simulink model "test_turb_sf9"  (R2013b)
settings: Solver=FixedStepDiscrete  StartTime=0.0  StopTime=15  FixedStep=0.005  RelTol=1e-3
libraries: simulink x1
settings Model: Creator=HSidaoui  LastModifiedBy=AGSilva
settings OptimizationCC: ExpressionDepthLimit=2147483647
settings DebuggingCC: StateNameClashWarn=warning

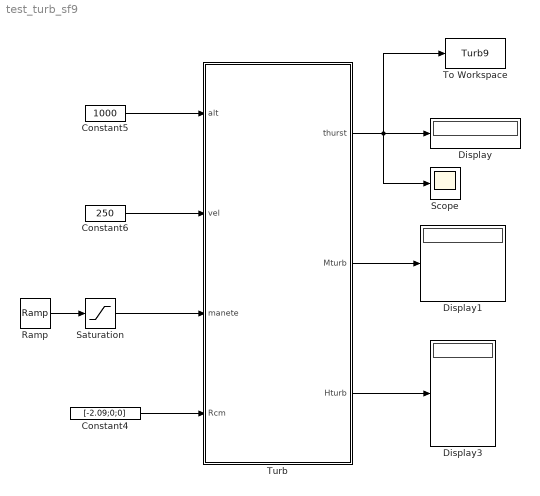
== system test_turb_sf9 ==
  Constant4 : Constant  Value=[-2.09;0;0]
  Constant5 : Constant  Value=1000
  Constant6 : Constant  Value=250
  Display : Display
  Display1 : Display
  Display3 : Display
  Ramp : simulink/Sources/Ramp  slope=0.1  start=0  X0=0
  Saturation : Saturate  UpperLimit=1  LowerLimit=0
  Scope : Scope
  To Workspace : ToWorkspace  VariableName=Turb9  SampleTime=-1  SaveFormat=Structure With Time
  Turb : Subsystem  TreatAsAtomicUnit=on
  wires:
  Constant5/1 -> Turb/1(alt)
  Turb/2(Mturb) -> Display1/1
  Turb/3(Hturb) -> Display3/1
  Constant6/1 -> Turb/2(vel)
  Constant4/1 -> Turb/4(Rcm)
  Ramp/1 -> Saturation/1
  Saturation/1 -> Turb/3(manete)
  Turb/1(thurst) -> Scope/1, To Workspace/1, Display/1

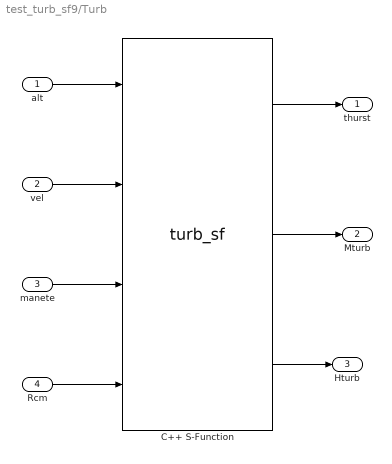
== system test_turb_sf9/Turb ==
  alt : Inport
  vel : Inport  Port=2
  manete : Inport  Port=3
  Rcm : Inport  Port=4
  C++ S-Function : S-Function  FunctionName=turb_sf  EnableBusSupport=off
  thurst : Outport
  Mturb : Outport  Port=2
  Hturb : Outport  Port=3
  wires:
  C++ S-Function/1 -> thurst/1
  alt/1 -> C++ S-Function/1
  vel/1 -> C++ S-Function/2
  manete/1 -> C++ S-Function/3
  Rcm/1 -> C++ S-Function/4
  C++ S-Function/2 -> Mturb/1
  C++ S-Function/3 -> Hturb/1
